simulink model "GA_PID_tuner"  (R2015a)
settings: Solver=ode45  StartTime=0.0  StopTime=1  RelTol=1e-3
settings Model: Creator=Shubham  LastModifiedBy=Shubham

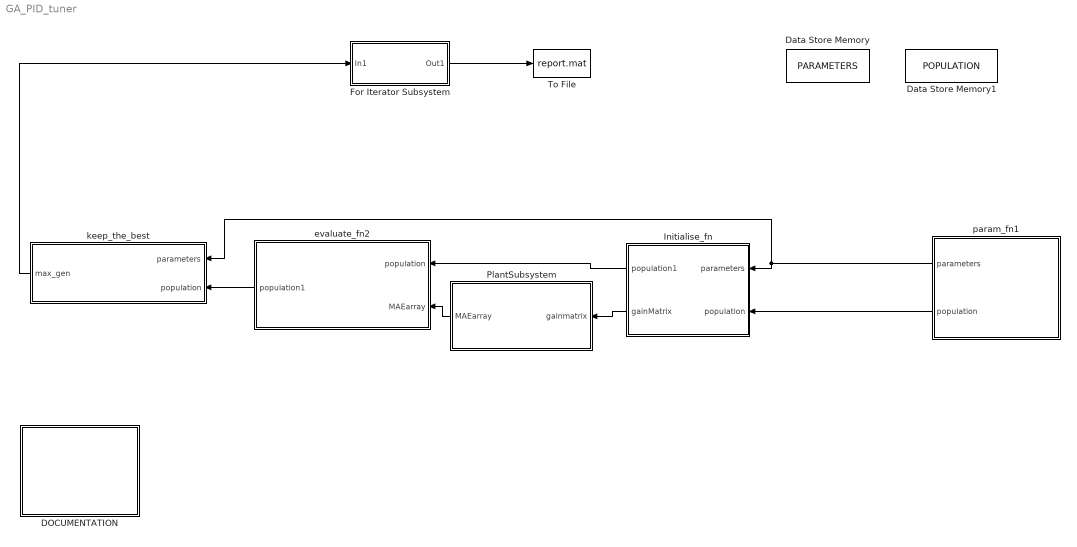
== system GA_PID_tuner ==
  "DOCUMENTATION " : MATLAB Function  TreatAsAtomicUnit=on
  Data Store Memory : DataStoreMemory  DataStoreName=PARAMETERS  InitialValue=[0 0 0 0 0 ]  OutDataTypeStr=double
  Data Store Memory1 : DataStoreMemory  DataStoreName=POPULATION  InitialValue=zeros(101,9)  OutDataTypeStr=double
  For Iterator Subsystem : Subsystem  TreatAsAtomicUnit=on
  Initialise_fn : MATLAB Function  TreatAsAtomicUnit=on
  PlantSubsystem : Subsystem
  To File : ToFile  Filename=report.mat  SampleTime=.1
  evaluate_fn2 : MATLAB Function  TreatAsAtomicUnit=on
  keep_the_best : MATLAB Function  TreatAsAtomicUnit=on
  param_fn1 : MATLAB Function  TreatAsAtomicUnit=on
  wires:
  param_fn1/1(parameters) -> Initialise_fn/1(parameters), keep_the_best/1(parameters)
  param_fn1/2(population) -> Initialise_fn/2(population)
  Initialise_fn/1(population1) -> evaluate_fn2/1(population)
  evaluate_fn2/1(population1) -> keep_the_best/2(population)
  keep_the_best/1(max_gen) -> For Iterator Subsystem/1(In1)
  For Iterator Subsystem/1(Out1) -> To File/1
  Initialise_fn/2(gainMatrix) -> PlantSubsystem/1(gainmatrix)
  PlantSubsystem/1(MAEarray) -> evaluate_fn2/2(MAEarray)

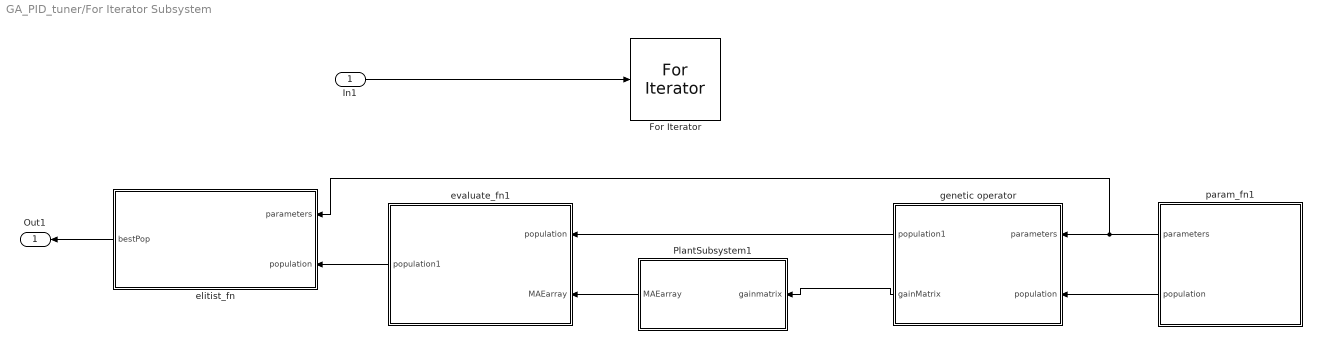
== system GA_PID_tuner/For Iterator Subsystem ==
  In1 : Inport
  For Iterator : ForIterator  ResetStates=reset  IterationSource=external  ShowIterationPort=off
  PlantSubsystem1 : Subsystem
  elitist_fn : MATLAB Function  TreatAsAtomicUnit=on
  evaluate_fn1 : MATLAB Function  TreatAsAtomicUnit=on
  genetic operator : MATLAB Function  TreatAsAtomicUnit=on
  param_fn1 : MATLAB Function  TreatAsAtomicUnit=on
  Out1 : Outport
  wires:
  genetic operator/1(population1) -> evaluate_fn1/1(population)
  evaluate_fn1/1(population1) -> elitist_fn/2(population)
  In1/1 -> For Iterator/1
  param_fn1/2(population) -> genetic operator/2(population)
  param_fn1/1(parameters) -> elitist_fn/1(parameters), genetic operator/1(parameters)
  genetic operator/2(gainMatrix) -> PlantSubsystem1/1(gainmatrix)
  PlantSubsystem1/1(MAEarray) -> evaluate_fn1/2(MAEarray)
  elitist_fn/1(bestPop) -> Out1/1

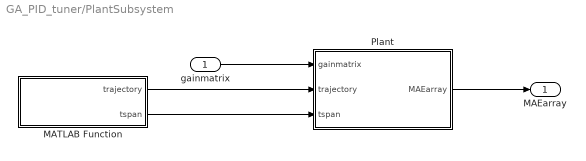
== system GA_PID_tuner/PlantSubsystem ==
  gainmatrix : Inport
  MATLAB Function : MATLAB Function  TreatAsAtomicUnit=on
  Plant : MATLAB Function  TreatAsAtomicUnit=on
  MAEarray : Outport
  wires:
  gainmatrix/1 -> Plant/1(gainmatrix)
  Plant/1(MAEarray) -> MAEarray/1
  MATLAB Function/1(trajectory) -> Plant/2(trajectory)
  MATLAB Function/2(tspan) -> Plant/3(tspan)

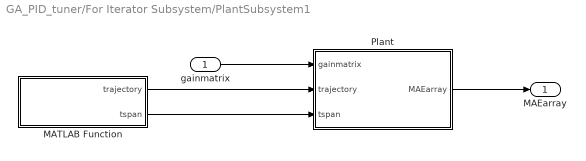
== system GA_PID_tuner/For Iterator Subsystem/PlantSubsystem1 ==
  gainmatrix : Inport
  MATLAB Function : MATLAB Function  TreatAsAtomicUnit=on
  Plant : MATLAB Function  TreatAsAtomicUnit=on
  MAEarray : Outport
  wires:
  gainmatrix/1 -> Plant/1(gainmatrix)
  Plant/1(MAEarray) -> MAEarray/1
  MATLAB Function/1(trajectory) -> Plant/2(trajectory)
  MATLAB Function/2(tspan) -> Plant/3(tspan)

== matlab function GA_PID_tuner/For Iterator Subsystem/param_fn1 ==
  data: parameters output size=[5 1]; population output size=[101 9]; PARAMETERS data_store_memory; POPULATION data_store_memory
function [parameters,population]= param_fn

global PARAMETERS;
global POPULATION;

parameters = PARAMETERS;
population = POPULATION;
end

== matlab function GA_PID_tuner/DOCUMENTATION  ==
function Documentation()

%1. In REPORT.MAT sample time can be set so that results are saved only for those time instants
%2. In FOR ITERATOR parameter " states when starting": reset: states are
%   reset prior to each time step 
% bounds for PID gains are defined twice: once in initialise() and another time in mutate() 






end

== matlab function GA_PID_tuner/Initialise_fn ==
  data: population1 output size=[101 9]; parameters input size=[5 1]; population input size=[101 9]; gainMatrix output size=[100 6]
function [population1,gainMatrix]= initialize (parameters,population)
%

% 
%  Purpose:
%
%    INITIALIZE initializes the genes within the variables bounds. 
%
% 

  
 
  
 
   kp_lb=0.01;
   kp_ub=10;
   kd_lb=0.01;
   kd_ub=10;
   ki_lb=.01;
   ki_ub=10;
   
   kp_dash_lb =0.01;
   kp_dash_ub =10;
   kd_dash_lb =0.01;
   kd_dash_ub =10;
   ki_dash_lb =.01;
   ki_dash_ub =10;

% 
%  Initialize variables within the bounds 
%
      
    
    for  j = 1:  parameters(1)
    
      
      population(j,1) = kp_lb + rand*(kp_ub-kp_lb);
      population(j,2) = kp_dash_lb + rand*(kp_dash_ub-kp_dash_lb);
      
      population(j,3) = kd_lb + rand*(kd_ub-kd_lb);
      population(j,4) = kd_dash_lb + rand*(kd_dash_ub-kd_dash_lb);
      
      population(j,5) = ki_lb + rand*(ki_ub-kp_lb);
      population(j,6) = ki_dash_lb + rand*(ki_dash_ub-ki_dash_lb);
      
    end
    
    population1 = population;
    
  % sending the gains corresponding to each member of the population  to plant
   gainMatrix = zeros(100,6);  
  %gainMatrix=zeros(parameters(1), parameters(3));
    for i=1 : parameters(1)
        for j=1:parameters(3)
        gainMatrix(i,j)=population(i,j);
        end
    end

end

== matlab function GA_PID_tuner/PlantSubsystem/MATLAB Function ==
  data: trajectory output; tspan output
function [trajectory,tspan] = traj()

tspan = 0:.01:5;
trajectory = zeros(length(tspan),6);

%% sinusoid
% for i =1:length(tspan)
% 
%     initial_pos = [0; 0];
%     v_max_y = 2;
%     a_max_y = 2;
% 
%     % Y
%     if tspan(i) <= v_max_y/a_max_y
%       dt = tspan(i);
%       acc_y = a_max_y;
%       vel_y = acc_y*dt;
%       pos_y = 0.5*acc_y*dt.^2;
%     elseif tspan(i) <= 2*v_max_y/a_max_y
%       dt = tspan(i) - v_max_y/a_max_y;
%       acc_y = 0;
%       vel_y = v_max_y;
%       pos_y = v_max_y.^2/(2*a_max_y) + v_max_y*dt;
%     elseif tspan(i) <= 3*v_max_y/a_max_y
%       dt = tspan(i) - 2*v_max_y/a_max_y;
%       acc_y = -a_max_y;
%       vel_y = v_max_y + acc_y*dt;
%       pos_y = 3*v_max_y.^2/(2*a_max_y) + v_max_y*dt + 0.5*acc_y*dt.^2;
%     else
%       acc_y = 0;
%       vel_y = 0;
%       pos_y = 2*v_max_y.^2/a_max_y;
%     end
% 
%     % Z
%     t_max = 3*v_max_y/a_max_y;
%     omega = 4*pi/t_max;
%     if tspan(i) < t_max
%       pos_z = 0.25*(1 - cos(omega*tspan(i)));
%       vel_z = 0.25*omega*sin(omega*tspan(i));
%       acc_z = 0.25*(omega.^2)*cos(omega*tspan(i));
%     else
%       pos_z = 0.25*(1 - cos(omega*t_max));
%       vel_z = 0;
%       acc_z = 0;
%     end
% 
% trajectory(i,1:2) = initial_pos + [pos_y; pos_z];
% trajectory(i,3:4) = [vel_y; vel_z];
% trajectory(i,5:6)= [acc_y; acc_z];
% 
% end

%% straight line
for i =1:length(tspan)

    initial_pos = [0; 1];
    v_max = 2;
    a_max = 2;

    if tspan(i) <= v_max/a_max
      dt = tspan(i);
      acc = [a_max; 0];
      vel = acc*dt;
      pos = 0.5*acc*dt.^2;
    elseif tspan(i) <= 2*v_max/a_max
      dt = tspan(i) - v_max/a_max;
      acc = [0; 0];
      vel = [v_max; 0];
      pos = [v_max.^2/(2*a_max);0] + [v_max*dt; 0];
    elseif tspan(i) <= 3*v_max/a_max
      dt = tspan(i) - 2*v_max/a_max;
      acc = [-a_max; 0];
      vel = [v_max; 0] + acc*dt;
      pos = [3*v_max.^2/(2*a_max); 0] + [v_max;0]*dt + 0.5*acc*dt.^2;
    else
      acc = [0;0];
      vel = [0;0];
      pos = [2*v_max.^2/a_max; 0];
   end

trajectory(i,1:2)  = initial_pos + pos;
trajectory(i,3:4)  = vel;
trajectory(i,5:6)  = acc;
end

end

== matlab function GA_PID_tuner/param_fn1 ==
  data: parameters output size=[5 1]; population output size=[101 9]
function [parameters,population]= param_fn()

%  Parameters:
%
%    MAXGENS is the maximum number of generations.
%
%    NVARS is the number of problem variables.
%
%    PMUTATION is the probability of mutation.
%
%    POPSIZE is the population size. 
%
%    PXOVER is the probability of crossover.                          
%
 parameters = zeros(5,1);
 parameters(1) = 100; % POPSIZE =20;
 parameters(2) = 100;% MAXGENS =100;
 parameters(3)= 6;   % NVARS =6;
 parameters(4) = 0.8; % PXOVER =0.8;
 parameters(5) = 0.15; % PMUTATION =0.15;


% population_i = ith member of the population
% population : n*m array; n= no of members in the population
  population = zeros(101 , 9);

% population.gene=[0 0 0 0 0 0 ];
% population.fitness=0;
% population.rfitness=0;
% population.cfitness=0;

% NOTE : IF CHANGES TO POPULATION SIZE OR NVARS IS MADE, MAKE NECESSARY 
% CHANGES IN "edit data"  


end

== matlab function GA_PID_tuner/evaluate_fn2 ==
  data: population input size=[101 9]; MAEarray input size=[100 1]; population1 output size=[101 9]
function population1 = evaluate_fn(population,MAEarray)


%****************************************************************************80
% 
%  Purpose:calculate fitness for each member of the population
%
%
%    
   [r, c] =size(MAEarray);
    for  i = 1:r
  
         population(i,7) = 1/(MAEarray(i)+.001);    
      
    end
    
    population1 = population;
end
  %****************************************************************************80

== matlab function GA_PID_tuner/For Iterator Subsystem/elitist_fn ==
  data: parameters input size=[5 1]; population input size=[101 9]; POPULATION data_store_memory; bestPop output size=[1 7]
function bestPop  = elitist (parameters,population)

%ELITIST


%****************************************************************************80
% 
%  Purpose:
%
%    ELITIST stores the best member of the previous generation.
%
%  Discussion:
%
%    The best member of the previous generation is stored as 
%    the last in the array. If the best member of the current 
%    generation is worse then the best member of the previous 
%    generation, the latter one would replace the worst member 
%    of the current population.
%

%  Local parameters:
%
%    Local,  BEST, the best fitness value.
%
%    Local,  WORST, the worst fitness value.
%

  
  
  best = population(1,7);
  worst = population(1,7);
  best_mem=0;
  worst_mem=0;
  
  for i =1: parameters(1) - 1
  
    if ( population(i+1,7) < population(i,7))
          if ( best <= population(i,7) )
               best = population(i,7);
               best_mem = i;
          end

          if ( population(i+1,7) <= worst )
               worst = population(i+1,7);
               worst_mem = i + 1;
          end

    
    else
          if ( population(i,7) <= worst )
               worst = population(i,7);
               worst_mem = i;
          end

          if ( best <= population(i+1,7) )
               best = population(i+1,7);
               best_mem = i + 1;
          end

    end    

  end
% 
%  If the best individual from the new population is better than 
%  the best individual from the previous population, then 
%  copy the best from the new population; else replace the 
%  worst individual from the current population with the 
%  best one from the previous generation                     
%
  if ( population(parameters(1)+1,7) <= best )
  
        for  i = 1:parameters(3)

          population(parameters(1)+1,i) = population(best_mem,i);
        end
          population(parameters(1)+1,7) = population(best_mem,7);

  else
  
        for  i = 1:parameters(3)

          population(worst_mem,i) = population(parameters(1)+1,i);
        end
          population(worst_mem,7) = population(parameters(1)+1,7);
        
  end
  
 global POPULATION;
 POPULATION = population; 
 bestPop =zeros(1,7);
 bestPop(1,1:6) = population(parameters(1)+1,1:6);
 bestPop(1,7) = population(parameters(1)+1,7);

end

== matlab function GA_PID_tuner/For Iterator Subsystem/evaluate_fn1 ==
  data: population input size=[101 9]; MAEarray input size=[100 1]; population1 output size=[101 9]
function population1 = evaluate_fn(population,MAEarray)


%****************************************************************************80
% 
%  Purpose:calculate fitness for each member of the population
%
%
%    
   
    [r, c] = size(MAEarray);
    for  mem = 1:r
  
    population(mem,7) = 1/(MAEarray(mem)+.001);    
      
    end
    
    population1 = population;
end
  %****************************************************************************80

== matlab function GA_PID_tuner/For Iterator Subsystem/genetic operator ==
  data: parameters input size=[5 1]; population input size=[101 9]; population1 output size=[101 9]; gainMatrix output size=[100 6]
function [population1,gainMatrix]  =genetic_operator(parameters,population)

 newpopulation = zeros(101 , 9);

%%
%SELECTOR FN
%****************************************************************************80
% 
%  Purpose:
%
%    SELECTOR is the selection function.
%
%  Discussion:
%
%    Standard proportional selection for maximization problems incorporating 
%    the elitist model.  This makes sure that the best member always survives.
%

%
% Find the total fitness of the population.
%
  sum = 0.0;
  for  i = 1: parameters(1)
       sum = sum + population(i,7);
  end
  
%
% Calculate the relative fitness of each member.
%
  for  i = 1: parameters(1)
        population(i,8) = population(i,7)/ sum;
  end
  
  
%
% Calculate the cumulative fitness.
%
  population(1,9) = population(1,8);
  
  for  i = 2:parameters(1)
      population(i,9) = population(i-1,9) +  population(i,8);
  end
  
%
% Select survivors using cumulative fitness. 
%
  for i = 1: parameters(1)
    p = rand; % generates a random no between 0 and 1
    if ( p < population(1,9) )
        newpopulation(i,:) = population(1,:);      
    
    else
        for j = 1: parameters(1)
            if ( population(j,9) <= p && p < population(j+1,9) )
                newpopulation(i,:) = population(j+1,:);
            end
        end
    end
  end
  
%
% Overwrite the old population with the new one.
%
  for  i = 1:parameters(1)
       population(i) = newpopulation(i); 
  end
 %*************************************************************************** 
  
 
 
 
  %%
 % CROSSOVER FN
  
%****************************************************************************80
% 
%  Purpose:
%
%    CROSSOVER selects two parents for the single point crossover.
%
%
%  Local parameters:
%
%    Local, int FIRST, is a count of the number of members chosen.
%
%  
  
  
  %rng(0,'twister');
  first=0; one=0;
  for  i = 1: parameters(1)
       x=  rand();
      if ( x < parameters(4) )
            first=first +1;
            if ( rem(first,2)==0)
                 
                %  Select the crossover point.
                %
                   point = 1+(parameters(3)-1)*rand;
                %
                %  Swap genes in positions 1 through POINT of one and i
                %
                    for  j = 1: point

                        t                 = population(one,j);
                        population(one,j) = population(i,j);
                        population(i,j)    = t;
                    end 
               
           else one = i;
           end
            
      end
  end
 %**************************************************************************
 
 
 
 

% MUTATE FN
 
 



%****************************************************************************80
% 
%  Purpose:
%
%    MUTATE performs a random uniform mutation. 
%
%  Discussion:
%
%    A variable selected for mutation is replaced by a random value 
%    between the lower and upper bounds of this variable.
%  
   
   
   
 
   kp_lb=0.01;
   kp_ub=10;
   kd_lb=0.01;
   kd_ub=10;
   ki_lb=.01;
   ki_ub=10;
   
   kp_dash_lb =0.01;
   kp_dash_ub =10;
   kd_dash_lb =0.01;
   kd_dash_ub =10;
   ki_dash_lb =.01;
   ki_dash_ub =10;

   
  
  for i = 1: parameters(1)
      for j=1 : parameters(3) 
          x = rand();
          if ( x < parameters(5) )
              switch (j)
              case 1 
                     population(i,1) = kp_lb + rand*(kp_ub-kp_lb);
              case 2 
                     population(i,2) = kp_dash_lb + rand*(kp_dash_ub-kp_dash_lb);        
              case 3 
                     population(i,3) = kd_lb + rand*(kd_ub-kd_lb);
              case 4 
                     population(i,4) = kd_dash_lb + rand*(kd_dash_ub-kd_dash_lb);
              case 5 
                     population(i,5) = ki_lb + rand*(ki_ub-kp_lb);
              case 6 
                     population(i,6) = ki_dash_lb + rand*(ki_dash_ub-ki_dash_lb); 
              end
          end
            
      end
  end
  
  
  
  


%****************************************************************************80

    % sending the gains corresponding to each member of the population  to plant
    gainMatrix=zeros(100,6);
    
    for i=1 : parameters(1)
        for j=1:parameters(3)
        gainMatrix(i,j)=population(i,j);
        end
    end

  population1 = population;
 end

== matlab function GA_PID_tuner/PlantSubsystem/Plant ==
  data: gainmatrix input size=[100 6]; MAEarray output size=[100 1]; trajectory input; tspan input
function MAEarray = plant(gainmatrix,trajectory,tspan)
%Calculating MAE based on the termination criteria set in 'simulation 2d.m'
% trajectory = Length(tspan)*6 matrix
params.gravity = 9.81;
params.mass = 0.18;
params.Ixx = 0.00025;
params.arm_length = 0.086;
params.minF = 0;
params.maxF = 2*.18*9.81;
dt = 0.01;
[popsize,~] = size(gainmatrix);
 MAEarray =zeros(popsize,1);

% State:
%[y; z; phi; y_dot; z_dot; phi_dot]

current_state = zeros(1,6);
desired_state = zeros(1,6);
% calculate MAE
%error =0.0;


% running  loop for all members of current generation
for j = 1:popsize

    current_state(1,:) = trajectory(1,:);
    desired_state(1,:) = trajectory(1,:);
    %error = error + abs(norm(current_state(1:2) - desired_state(1:2)))+
    
    Kp_z =gainmatrix(j,1);
    Kd_z = gainmatrix(j,2);
    Kp_y = gainmatrix(j,3);
    Kd_y = gainmatrix(j,4);
    Kp_a =gainmatrix(j,5) ;
    Kd_a = gainmatrix(j,6);
        
    for i = 2: length(tspan)
        
        
      % CONTROLLER FUNCTION to get F and M
        desired_state(1,:) = trajectory(i,:);
        
        F = params.mass*(params.gravity + desired_state(6) + Kd_z*(desired_state(4)-current_state(4)) + Kp_z*(desired_state(2))-current_state(2));
        phi_c = -(1/params.gravity)*(desired_state(5) + Kd_y*(desired_state(3)-current_state(3) + Kp_y*(desired_state(1)-current_state(1))));
        phi_c_dot = 0;
        phi_c_2dot = 0;
        M = params.Ixx*(phi_c_2dot + Kd_a*(phi_c_dot-current_state(6)) + Kp_a*(phi_c-current_state(3)));

        
        
      % SYS_EOM FUNCTION to get new current_state
       
        u1 = 0.5*(F - M/params.arm_length);
        u2 = 0.5*(F + M/params.arm_length);

        u1_clamped = min(max(params.minF/2, u1), params.maxF/2);
        u2_clamped = min(max(params.minF/2, u2), params.maxF/2);
        F_clamped = u1_clamped + u2_clamped;
        M_clamped = (u2_clamped - u1_clamped)*params.arm_length;

        
        sdot = [current_state(4);
                current_state(5);
                current_state(6);
                -F_clamped*sin(current_state(3))/params.mass;
                F_clamped*cos(current_state(3))/params.mass - params.gravity;
                M_clamped/params.Ixx]';


        temp = current_state + sdot*dt;
        current_state = temp;
     
    end
    desired_state = trajectory(end,:);
    MAEarray(j) = norm( current_state(1:2) - desired_state(1:2) )+ ( norm( current_state(4:5) ) )...
                   + abs( current_state(3) );
    
end

end

== matlab function GA_PID_tuner/keep_the_best ==
  data: parameters input size=[5 1]; population input size=[101 9]; PARAMETERS data_store_memory; POPULATION data_store_memory; max_gen output
function max_gen = keep_the_best (parameters,population)


%****************************************************************************80
% 
%  Purpose:
%
%    KEEP_THE_BEST keeps track of the best member of the population. 
%
%  Discussion:
%
%    Note that the last entry in the array Population holds a 
%    copy of the best individual.
%  Local parameters:
%
%    Local,  CUR_BEST, the index of the best individual.
%  
   
 %  next_i = 1;
   cur_best=0;
  
   population(parameters(1),7)=0;
   
    for i = 1: parameters(1)
  
    if ( population(parameters(1)+1,7) < population(i,7) )
         cur_best = i;
         population(parameters(1)+1,7) = population(i,7);
    end
    end
% 
%  Once the best member in the population is found, copy the genes.
%
    for  i = 1: parameters(3)
  
      population(parameters(1)+1,:) = population(cur_best,:);
    end
    
    
global PARAMETERS;
global POPULATION;
PARAMETERS =  parameters;
POPULATION = population;

max_gen =5000;


end

== matlab function GA_PID_tuner/For Iterator Subsystem/PlantSubsystem1/MATLAB Function ==
  data: trajectory output; tspan output
function [trajectory,tspan] = traj()

tspan = 0:.01:5;
trajectory = zeros(length(tspan),6);

%% sinusoid
% for i =1:length(tspan)
% 
%     initial_pos = [0; 0];
%     v_max_y = 2;
%     a_max_y = 2;
% 
%     % Y
%     if tspan(i) <= v_max_y/a_max_y
%       dt = tspan(i);
%       acc_y = a_max_y;
%       vel_y = acc_y*dt;
%       pos_y = 0.5*acc_y*dt.^2;
%     elseif tspan(i) <= 2*v_max_y/a_max_y
%       dt = tspan(i) - v_max_y/a_max_y;
%       acc_y = 0;
%       vel_y = v_max_y;
%       pos_y = v_max_y.^2/(2*a_max_y) + v_max_y*dt;
%     elseif tspan(i) <= 3*v_max_y/a_max_y
%       dt = tspan(i) - 2*v_max_y/a_max_y;
%       acc_y = -a_max_y;
%       vel_y = v_max_y + acc_y*dt;
%       pos_y = 3*v_max_y.^2/(2*a_max_y) + v_max_y*dt + 0.5*acc_y*dt.^2;
%     else
%       acc_y = 0;
%       vel_y = 0;
%       pos_y = 2*v_max_y.^2/a_max_y;
%     end
% 
%     % Z
%     t_max = 3*v_max_y/a_max_y;
%     omega = 4*pi/t_max;
%     if tspan(i) < t_max
%       pos_z = 0.25*(1 - cos(omega*tspan(i)));
%       vel_z = 0.25*omega*sin(omega*tspan(i));
%       acc_z = 0.25*(omega.^2)*cos(omega*tspan(i));
%     else
%       pos_z = 0.25*(1 - cos(omega*t_max));
%       vel_z = 0;
%       acc_z = 0;
%     end
% 
% trajectory(i,1:2) = initial_pos + [pos_y; pos_z];
% trajectory(i,3:4) = [vel_y; vel_z];
% trajectory(i,5:6)= [acc_y; acc_z];
% 
% end

%% straight line
for i =1:length(tspan)

    initial_pos = [0; 1];
    v_max = 2;
    a_max = 2;

    if tspan(i) <= v_max/a_max
      dt = tspan(i);
      acc = [a_max; 0];
      vel = acc*dt;
      pos = 0.5*acc*dt.^2;
    elseif tspan(i) <= 2*v_max/a_max
      dt = tspan(i) - v_max/a_max;
      acc = [0; 0];
      vel = [v_max; 0];
      pos = [v_max.^2/(2*a_max);0] + [v_max*dt; 0];
    elseif tspan(i) <= 3*v_max/a_max
      dt = tspan(i) - 2*v_max/a_max;
      acc = [-a_max; 0];
      vel = [v_max; 0] + acc*dt;
      pos = [3*v_max.^2/(2*a_max); 0] + [v_max;0]*dt + 0.5*acc*dt.^2;
    else
      acc = [0;0];
      vel = [0;0];
      pos = [2*v_max.^2/a_max; 0];
   end

trajectory(i,1:2)  = initial_pos + pos;
trajectory(i,3:4)  = vel;
trajectory(i,5:6)  = acc;
end

end

== matlab function GA_PID_tuner/For Iterator Subsystem/PlantSubsystem1/Plant ==
  data: gainmatrix input size=[100 6]; MAEarray output size=[100 1]; trajectory input; tspan input
function MAEarray = plant(gainmatrix,trajectory,tspan)
%Calculating MAE based on the termination criteria set in 'simulation 2d.m'
% trajectory = Length(tspan)*6 matrix
params.gravity = 9.81;
params.mass = 0.18;
params.Ixx = 0.00025;
params.arm_length = 0.086;
params.minF = 0;
params.maxF = 2*.18*9.81;
dt = 0.01;
[popsize,~] = size(gainmatrix);
 MAEarray =zeros(popsize,1);

% State:
%[y; z; phi; y_dot; z_dot; phi_dot]

current_state = zeros(1,6);
desired_state = zeros(1,6);
% calculate MAE
%error =0.0;


for j = 1:popsize

    current_state(1,:) = trajectory(1,:);
    desired_state(1,:) = trajectory(1,:);
    %error = error + abs(norm(current_state(1:2) - desired_state(1:2)))+
    
    for i = 2: length(tspan)
        
      % CONTROLLER FUNCTION to get F and M
        desired_state(1,:) = trajectory(i,:);
        Kp_z =gainmatrix(j,1);
        Kd_z = gainmatrix(j,2);
        Kp_y = gainmatrix(j,3);
        Kd_y = gainmatrix(j,4);
        Kp_a =gainmatrix(j,5) ;
        Kd_a = gainmatrix(j,6);

        

        F = params.mass*(params.gravity + desired_state(6) + Kd_z*(desired_state(4)-current_state(4)) + Kp_z*(desired_state(2))-current_state(2));
        phi_c = -(1/params.gravity)*(desired_state(5) + Kd_y*(desired_state(3)-current_state(3) + Kp_y*(desired_state(1)-current_state(1))));
        phi_c_dot = 0;
        phi_c_2dot = 0;
        M = params.Ixx*(phi_c_2dot + Kd_a*(phi_c_dot-current_state(6)) + Kp_a*(phi_c-current_state(3)));

        
        
      % SYS_EOM FUNCTION to get new current_state
       
        u1 = 0.5*(F - M/params.arm_length);
        u2 = 0.5*(F + M/params.arm_length);

        u1_clamped = min(max(params.minF/2, u1), params.maxF/2);
        u2_clamped = min(max(params.minF/2, u2), params.maxF/2);
        F_clamped = u1_clamped + u2_clamped;
        M_clamped = (u2_clamped - u1_clamped)*params.arm_length;

        
        sdot = [current_state(4);
                current_state(5);
                current_state(6);
                -F_clamped*sin(current_state(3))/params.mass;
                F_clamped*cos(current_state(3))/params.mass - params.gravity;
                M_clamped/params.Ixx]';


        temp = current_state + sdot*dt;
        current_state = temp;
      % calculating MAE using error in pos
      %  error = error + abs(norm(current_state(1:2) - desired_state(1:2)));
    end
    
    MAEarray(j) = norm( current_state(1:2) - desired_state(1:2) )+ ( norm( current_state(4:5) ) )...
                   + abs( current_state(3) );
    
end

end
